simulink model "TBRe_Mod"  (R2017b)
settings: Solver=FixedStepDiscrete  StartTime=0.0  StopTime=inf  FixedStep=0.0001  RelTol=1e-3
PostLoadFcn:
  | model_init();
values from neighbouring files (symbols this model uses):
  SOC_Calc_bPoint = Simulink.Parameter    [ecuparams.m]
  SOC_Calc_Data = Simulink.Parameter    [ecuparams.m]
  Voltage_Act_bPoint = Simulink.Parameter    [ecuparams.m]
  Voltage_Act_Data = Simulink.Parameter    [ecuparams.m]
undefined symbols (not defined in the file or in its folder): _240Nm_Breakpoint, _240Nm_Data, Brake_Active_Threshold, Brk1_OOR_High, Brk1_OOR_Low, Brk2_OOR_High, Brk2_OOR_Low, Motor_To_Road_Speed_Ratio, Throttle_Active_Threshold, Throttle_Torque_Map_
libraries: simulink x26
(part 5 of 8)

== system TBRe_Mod/MainTask/Pre_Processing_Layer/Pedal_Box ==
  note: Non hysteresis brake and throttle bools
  note: Throttle bool and Brake bool are arbitrary values (not rules)
  note: Overall Functionality:
      | - All pedal box sensor values are checked to ensure that they are in the correct voltage range
      | - These sensors are then scaled to be between 0-100 %
      | - APPS Implausibility is performed
      | - Brake pedal implausibility is performed
      | - Thresholds for when brake is considered active, and throttle is considered active are set here (used for RTD and Brake Light activation respectively)
  DAL_Data : Inport
  APPS and BP Plausibility : Subsystem
  APPS_Implausibility_Check : Subsystem
  BPPS_Implausibility_Check : Subsystem
  Brake Bool Hysteresis : Relay  OnSwitchValue=Brake_Active_Threshold  OffSwitchValue=Brake_Active_Threshold/2  OutDataTypeStr=boolean
  Brake Out Of Range Check : Subsystem
  Bus Creator : BusCreator  Inputs=13
  Bus Selector : BusSelector  OutputSignals=DAL_Hardwired.Throttle1_Voltage,DAL_Hardwired.Throttle2_Voltage,DAL_Hardwired.Brake1_Pressure,DAL_Hardwired.Brake2_Pressure
  Memory read : S-Function  Commented=on  FunctionName=NsiMem_Read  Parameters=name_var,type_var,size_var,tunable_var  SFunctionDeploymentMode=off  EnableBusSupport=off  mask(Memory read){name_var=Gearing_Ratio, type_var=Unsigned Byte, size_var=1, tunable_var=on}
      mask prompts: name_var "Variable name :"; type_var "Type :"; size_var "Dim of table :"; tunable_var "Is Tunable By USB?"
      mask help: Reads current value of variable memory declared in the configurator block in calibration page.
      mask init:
      | NsiMem_Read_InitializationFcn();
      settings: OpenFcn=NsiMem_Read_OpenFcn();
      mask Help:
      | eval('block=get_param(gcb, ''RTWdata'');')
      | web([docroot '\toolbox\MUXlink\html\blocks/' block.MUXlink_BlockType '.html'])
      mask TypeOptions name_var: Gearing_Ratio | Wheel_Size | Brake1_High | Brake2_High | Throttle1_High | Throttle2_High | Brake1_Low | Brake2_Low | Throttle1_Low | Throttle2_Low | Max_Torque_Std | Green_TSAL2 | Green_TSAL1 | Max_Torque_Boost | MCU_Ignition | LV_Low_Voltage_Warning | MCUMotor_Temp_Warning | Target_Slip_Ratio | TC_P_Gain | MinTC_Torque | Max_Regen | INV_Torque_limit | INV_Speed_Limit_Fwd | INV_Speed_limit_Rev | INV_DC_Link_Target | INV_DC_Link_Regen_Imax | INV_DC_Link_Discharge_Imax | INV_Regen_Torque_Limit | INV_Id_Debug | INV_Iq_debug | Init_System_Start | Init_System_end | Brake1_Pressure_Scaling | Brake2_Pressure_Scaling | Regen_Coast
      mask Callback name_var: NsiMem_Read_ApplyFcn(1);
      mask TypeOptions type_var: Boolean | Signed Byte | Unsigned Byte | Signed Word | Unsigned Word | Signed Double Word | Unsigned Double Word | Single Float | Double Float
      mask Callback type_var: NsiMem_Read_ApplyFcn(2);
      mask Callback size_var: NsiMem_Read_ApplyFcn(3);
      mask Callback tunable_var: NsiMem_Read_ApplyFcn(4);
      mask Display: image(imread('nsi.bmp'));text(0.5, 0.35, 'Gearing_Ratio', 'horizontalAlignment', 'center', 'verticalAlignment', 'base');plot([0.05 0.05 0.05 0.05 0.05 0.05 0.05 0.05 0.05 0.05]);port_label('output', 1, 'Read');
  Memory read1 : S-Function  Commented=on  FunctionName=NsiMem_Read  Parameters=name_var,type_var,size_var,tunable_var  SFunctionDeploymentMode=off  EnableBusSupport=off  mask(Memory read){name_var=Gearing_Ratio, type_var=Unsigned Byte, size_var=1, tunable_var=on}
      mask prompts: name_var "Variable name :"; type_var "Type :"; size_var "Dim of table :"; tunable_var "Is Tunable By USB?"
      mask help: Reads current value of variable memory declared in the configurator block in calibration page.
      mask init:
      | NsiMem_Read_InitializationFcn();
      settings: OpenFcn=NsiMem_Read_OpenFcn();
      mask Help:
      | eval('block=get_param(gcb, ''RTWdata'');')
      | web([docroot '\toolbox\MUXlink\html\blocks/' block.MUXlink_BlockType '.html'])
      mask TypeOptions name_var: Gearing_Ratio | Wheel_Size | Brake1_High | Brake2_High | Throttle1_High | Throttle2_High | Brake1_Low | Brake2_Low | Throttle1_Low | Throttle2_Low | Max_Torque_Std | Green_TSAL2 | Green_TSAL1 | Max_Torque_Boost | MCU_Ignition | LV_Low_Voltage_Warning | MCUMotor_Temp_Warning | Target_Slip_Ratio | TC_P_Gain | MinTC_Torque | Max_Regen | INV_Torque_limit | INV_Speed_Limit_Fwd | INV_Speed_limit_Rev | INV_DC_Link_Target | INV_DC_Link_Regen_Imax | INV_DC_Link_Discharge_Imax | INV_Regen_Torque_Limit | INV_Id_Debug | INV_Iq_debug | Init_System_Start | Init_System_end | Brake1_Pressure_Scaling | Brake2_Pressure_Scaling | Regen_Coast
      mask Callback name_var: NsiMem_Read_ApplyFcn(1);
      mask TypeOptions type_var: Boolean | Signed Byte | Unsigned Byte | Signed Word | Unsigned Word | Signed Double Word | Unsigned Double Word | Single Float | Double Float
      mask Callback type_var: NsiMem_Read_ApplyFcn(2);
      mask Callback size_var: NsiMem_Read_ApplyFcn(3);
      mask Callback tunable_var: NsiMem_Read_ApplyFcn(4);
      mask Display: image(imread('nsi.bmp'));text(0.5, 0.35, 'Gearing_Ratio', 'horizontalAlignment', 'center', 'verticalAlignment', 'base');plot([0.05 0.05 0.05 0.05 0.05 0.05 0.05 0.05 0.05 0.05]);port_label('output', 1, 'Read');
  Relational Operator : RelationalOperator  Commented=on  OutDataTypeStr=boolean  RndMeth=Simplest
  Relational Operator1 : RelationalOperator  Commented=on  OutDataTypeStr=boolean  RndMeth=Simplest
  Sensor Plausibility : Subsystem
  Throttle Bool Hysteresis : Relay  OnSwitchValue=Throttle_Active_Threshold  OffSwitchValue=Throttle_Active_Threshold/2  OutDataTypeStr=boolean
  Voltage_to_% Conversion : Subsystem
  Pedal_Box_Data : Outport
  wires:
  Bus Creator/1 -> Pedal_Box_Data/1
  DAL_Data/1 -> Brake Out Of Range Check/1(Brake Voltages), Bus Selector/1
  Voltage_to_% Conversion/1(T1%) -> Bus Creator/2, APPS_Implausibility_Check/1(Throttle1_Per)  "Throttle1_Per"
  Voltage_to_% Conversion/2(T2%) -> Bus Creator/3, APPS_Implausibility_Check/2(Throttle2_Per)  "Throttle2_Per"
  Throttle Bool Hysteresis/1 -> Bus Creator/6  "Throttle_Bool"
  Brake Bool Hysteresis/1 -> Bus Creator/8  "Brake_Bool"
  APPS and BP Plausibility/1(Throttle_%) -> Bus Creator/5, Throttle Bool Hysteresis/1  "Throttle_Percentage"
  APPS and BP Plausibility/2(APPS_BP_Implausibility) -> Bus Creator/7  "APPS_BP_Implausibility"
  APPS_Implausibility_Check/1(APPS_Implausibility) -> Bus Creator/4  "APPS_Implausibility"
  APPS_Implausibility_Check/2(Throttle_%) -> APPS and BP Plausibility/1(Throttle_In)
  Sensor Plausibility/1(Pedal_Sensor_Fail) -> Bus Creator/1  "Pedal_Sensor_Fail"
  Bus Selector/1 -> Sensor Plausibility/1(<Throttle1_Voltage>)  "<Throttle1_Voltage>"
  Bus Selector/2 -> Sensor Plausibility/2(<Throttle2_Voltage>)  "<Throttle2_Voltage>"
  Sensor Plausibility/2(TV1_Out) -> Voltage_to_% Conversion/1(Throttle1)
  Sensor Plausibility/3(TV2_Out) -> Voltage_to_% Conversion/2(Throttle2)
  Bus Selector/3 -> Sensor Plausibility/3(<Brake_Voltage>1)  "<Brake1_Pressure>"
  Bus Selector/4 -> Sensor Plausibility/4(<Brake_Voltage>2)  "<Brake2_Pressure>"
  Sensor Plausibility/4(BV1_Out) -> Voltage_to_% Conversion/3(BrakePress1)
  Sensor Plausibility/5(BV1_Out1) -> Voltage_to_% Conversion/4(BrakePress2)
  BPPS_Implausibility_Check/1(Brake_%) -> Brake Bool Hysteresis/1, Bus Creator/9, APPS and BP Plausibility/2(Brake_%)  "Brake_Percentage"
  BPPS_Implausibility_Check/2(BPPS_Implausibility) -> Bus Creator/10  "BPPS_Implausibility"
  Voltage_to_% Conversion/3(BPr%1) -> Bus Creator/11, BPPS_Implausibility_Check/1(Brake1_Per)  "Brake1_Per"
  Voltage_to_% Conversion/4(BPr%2) -> Bus Creator/12, BPPS_Implausibility_Check/2(Brake2_Per)  "Brake2_Per"
  ? -> Relational Operator/1  "Brake_Percentage"
  Memory read1/1 -> Relational Operator/2
  ? -> Relational Operator1/1  "Throttle_Percentage"
  Memory read/1 -> Relational Operator1/2
  Brake Out Of Range Check/1(Brake Out Of Range) -> Bus Creator/13  "Brake_OOR"

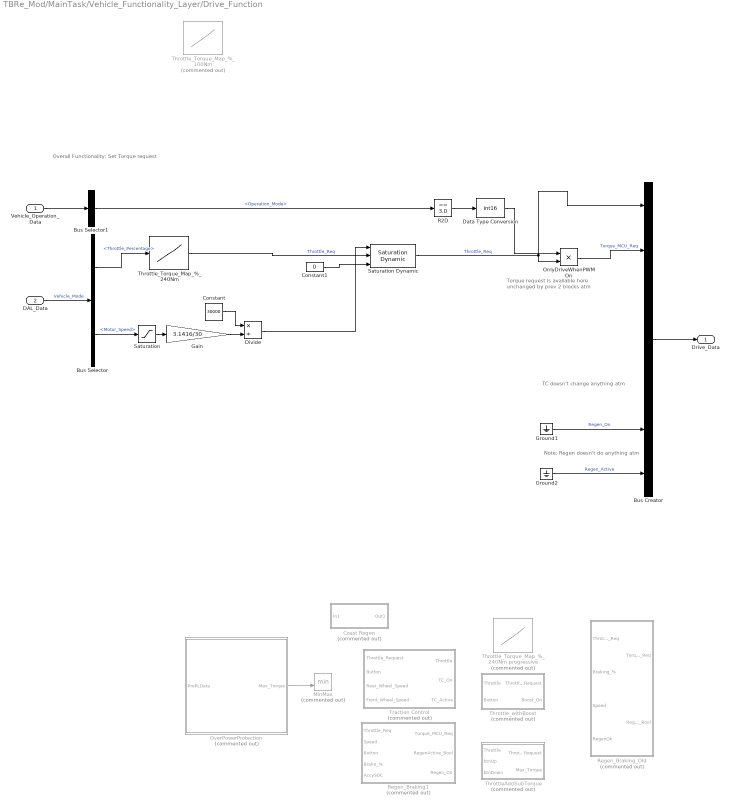
== system TBRe_Mod/MainTask/Vehicle_Functionality_Layer/Drive_Function ==
  note: Torque request is available here
      | unchanged by prev 2 blocks atm
  note: TC doesn't change anything atm
  note: Note: Regen doesn't do anything atm
  note: Overall Functionality:
      | Set Torque request
  Vehicle_Operation_Data : Inport
  DAL_Data : Inport  Port=2
  Bus Creator : BusCreator  Inputs=7
  Bus Selector : BusSelector  OutputSignals=Pedal_Box_Data.Throttle_Percentage,HAL_Data.DAL_CAN.DAL_MCUCAN.Motor_Speed
  Bus Selector1 : BusSelector  OutputSignals=Operation_Mode
  Coast Regen : Subsystem  Commented=on
  Constant : Constant  Value=30000
  Constant1 : Constant  Value=0
  Data Type Conversion : DataTypeConversion  OutDataTypeStr=int16
  Divide : Product  Inputs=*/
  Gain : Gain  Gain=3.1416/30
  Ground1 : Ground
  Ground2 : Ground
  MinMax : MinMax  Commented=on  Inputs=2
  OnlyDriveWhenPWMOn : Product  OutDataTypeStr=int16
  OverPowerProtection : Subsystem  Commented=on
  R2D : simulink/Logic and Bit Operations/Compare To Constant  relop===  const=3.0  OutDataTypeStr=boolean
  Regen_Braking1 : Subsystem  Commented=on
  Regen_Braking_Old : Subsystem  Commented=on
  Saturation : Saturate  UpperLimit=10000  LowerLimit=1
  Saturation Dynamic : simulink/Discontinuities/Saturation Dynamic  OutMin=[]  OutMax=[]  OutDataTypeStr=Inherit: Same as second input  OutDataType=fixdt(1, 16)  OutScaling=2^-10  DoSatur=off
  ThrottleAddSubTorque : Subsystem  Commented=on
  Throttle_Torque_Map_%_100Nm : Lookup_n-D  Commented=on  NumberOfTableDimensions=1  BreakpointsForDimension1=[0,25,100]  Table=[0,10,100]  ExtrapMethod=Clip  UseLastTableValue=on  InternalRulePriority=Speed  OutDataTypeStr=int16  RndMeth=Simplest  InputSameDT=on
  Throttle_Torque_Map_%_240Nm : Lookup_n-D  NumberOfTableDimensions=1  BreakpointsForDimension1=Throttle_Torque_Map_%_240Nm_Breakpoint  Table=Throttle_Torque_Map_%_240Nm_Data  ExtrapMethod=Clip  UseLastTableValue=on  InternalRulePriority=Speed  OutDataTypeStr=int16  RndMeth=Simplest  InputSameDT=on
  Throttle_Torque_Map_%_240Nm progressive : Lookup_n-D  Commented=on  NumberOfTableDimensions=1  BreakpointsForDimension1=[0,10,20,40,60,80,100]  Table=[0,20,30,50,120,200,240]  ExtrapMethod=Clip  UseLastTableValue=on  InternalRulePriority=Speed  OutDataTypeStr=int16  RndMeth=Simplest  InputSameDT=on
  Throttle_withBoost : Subsystem  Commented=on
  Traction Control : Subsystem  Commented=on
  Drive_Data : Outport
  wires:
  Bus Selector1/1 -> R2D/1  "<Operation_Mode>"
  Bus Selector/1 -> Throttle_Torque_Map_%_240Nm/1  "<Throttle_Percentage>"
  R2D/1 -> Data Type Conversion/1
  Vehicle_Operation_Data/1 -> Bus Selector1/1
  DAL_Data/1 -> Bus Selector/1  "Vehicle_Mode"
  OnlyDriveWhenPWMOn/1 -> Bus Creator/2  "Torque_MCU_Req"
  Bus Creator/1 -> Drive_Data/1
  Data Type Conversion/1 -> OnlyDriveWhenPWMOn/1
  Ground1/1 -> Bus Creator/6  "Regen_On"
  OverPowerProtection/1(Max_Torque) -> MinMax/2
  Ground2/1 -> Bus Creator/7  "Regen_Active"
  Saturation Dynamic/1 -> Bus Creator/1, OnlyDriveWhenPWMOn/2  "Throttle_Req"
  Bus Selector/2 -> Saturation/1  "<Motor_Speed>"
  Throttle_Torque_Map_%_240Nm/1 -> Saturation Dynamic/2  "Throttle_Req"
  Gain/1 -> Divide/2
  Constant/1 -> Divide/1
  Divide/1 -> Saturation Dynamic/1
  Constant1/1 -> Saturation Dynamic/3
  Saturation/1 -> Gain/1

== system TBRe_Mod/MainTask/Vehicle_Functionality_Layer/Vehicle_Operation_Mode ==
  note: Checks high contactor has physically closed and request to close is beening sent
  note: System_Error
  note: Overall Functionality:
      | Vehicle state machine for Ready to drive after checking the vehicle is safe,
      | Put vehicel in error state if nessassery
      | Activate TSS
  PrePL_Data : Inport
  Bus Creator : BusCreator  Inputs=6
  Bus Selector1 : BusSelector  OutputSignals=Pedal_Box_Data.Throttle_Bool,Pedal_Box_Data.Brake_Bool,Buttons.btnRTD,HAL_Data.DAL_Hardwired.AIRHigh
  Bus Selector2 : BusSelector  OutputSignals=HAL_Data.DAL_CAN.DAL_SENSORCAN.Shutdown_Error,LV_Battery.LV_Warning,MCU_Temps_Data.MCU_Motor_Temp_Error,Pedal_Box_Data.Brake_OOR,IMD_Data.IMD_Freq
  Bus Selector3 : BusSelector  OutputSignals=HAL_Data.DAL_Hardwired.btnPreCharge_Input,HAL_Data.DAL_Hardwired.AIRLow,HAL_Data.DAL_Hardwired.Latch_Status
  Compare To Constant2 : simulink/Logic and Bit Operations/Compare To Constant  relop=~=  const=0  OutDataTypeStr=boolean
  Logical Operator1 : Logic  AllPortsSameDT=off  OutDataTypeStr=boolean
  Logical Operator2 : Logic  AllPortsSameDT=off  OutDataTypeStr=boolean
  Operaton_Mode : Stateflow chart  TreatAsAtomicUnit=on
  TS Enable : Stateflow chart  TreatAsAtomicUnit=on
  TSS (Precharge Finisher) : Subsystem
  Terminator{1,3..5} (4 alike) : Terminator
  VOM_Data : Outport
  wires:
  Bus Selector1/2 -> Operaton_Mode/2(Brake)  "<Brake_Bool>"
  Logical Operator1/1 -> Bus Creator/3  "ECU_Ok"
  Operaton_Mode/1(Control_Word) -> Bus Creator/1  "Control_Word"
  Operaton_Mode/2(State) -> Compare To Constant2/1, Bus Creator/2  "Operation_Mode"
  Bus Creator/1 -> VOM_Data/1  "Vehicle_Operation_Data"
  Bus Selector1/1 -> Operaton_Mode/1(Throttle)  "<Throttle_Bool>"
  TSS (Precharge Finisher)/1(TS_StartUp) -> Logical Operator2/2, Bus Creator/4  "TSS"
  Bus Selector1/3 -> Operaton_Mode/3(btnRTD)  "<btnRTD>"
  Bus Selector2/3 -> Terminator3/1  "<MCU_Motor_Temp_Error>"
  Bus Selector2/2 -> Terminator5/1  "<LV_Warning>"
  Bus Selector2/1 -> Terminator4/1  "<Shutdown_Error>"
  PrePL_Data/1 -> Bus Selector3/1, TSS (Precharge Finisher)/1(PrePL_Data), Bus Selector2/1, Bus Selector1/1  "Input_Data"
  Bus Selector3/1 -> TS Enable/1(btnPreCharge)  "<btnPreCharge_Input>"
  Bus Selector3/2 -> TS Enable/2(LowAIR_Status)  "<AIRLow>"
  TS Enable/1(TS_Enable) -> Logical Operator1/2, TSS (Precharge Finisher)/2(TS_Enable)
  Compare To Constant2/1 -> Logical Operator1/1
  Bus Selector1/4 -> Logical Operator2/1  "<AIRHigh>"
  TS Enable/2(State) -> Bus Creator/5  "TS_Enable_State"
  Logical Operator2/1 -> Operaton_Mode/5(Discharge_ready)
  Bus Selector3/3 -> TS Enable/4(Latch_Status)  "<Latch_Status>"
  Bus Selector2/4 -> Terminator1/1  "<Brake_OOR>"
  ? -> Bus Creator/6  "Reset_Out"

== system TBRe_Mod/MainTask/Comms_And_Data_Acquisition_Layer/Hardwired_Inputs_2019/AIRs ==
  DigitalInput : S-Function  FunctionName=NsiIo_DigitalInput  Parameters=channel,is_trigger,typeof_trigger,is_wakeup,wakeup_level  SFunctionDeploymentMode=off  EnableBusSupport=off  mask(MUXlink I/O Digital Input){channel=21, is_trigger=off, typeof_trigger=Either, is_wakeup=off, wakeup_level=Low level}
      mask prompts: channel "Channel ?"; is_trigger "Trigger ?"; typeof_trigger "Type of Trigger ?"; is_wakeup "Wake-up ?"; wakeup_level "Wake-up level ?"
      mask help: Read digital input from I/O channel.
      mask init:
      | NsiIo_DigitalInput_InitializationFcn();
      settings: OpenFcn=NsiIo_DigitalInput_OpenFcn();
      mask Help:
      | eval('block=get_param(gcb, ''RTWdata'');')
      | web([docroot '\toolbox\MUXlink\html\blocks/' block.MUXlink_BlockType '.html'])
      mask Callback channel: NsiIo_DigitalInput_ApplyFcn(1);
      mask Callback is_trigger: NsiIo_DigitalInput_ApplyFcn(2);
      mask TypeOptions typeof_trigger: Rising | Falling | Either
      mask Callback typeof_trigger: NsiIo_DigitalInput_ApplyFcn(3);
      mask Callback is_wakeup: NsiIo_DigitalInput_ApplyFcn(4);
      mask TypeOptions wakeup_level: Low level | High level
      mask Callback wakeup_level: NsiIo_DigitalInput_ApplyFcn(5);
      mask Display: image(imread('nsi.bmp'));text(0.5, 0.2, 'DigitalInput_21', 'horizontalAlignment', 'center', 'verticalAlignment', 'base');plot([0.05 0.05 0.05 0.05 0.05 0.05 0.05 0.05 0.05 0.05]);port_label('output', 1, 'Battery : F1');
  DigitalInput5 : S-Function  FunctionName=NsiIo_DigitalInput  Parameters=channel,is_trigger,typeof_trigger,is_wakeup,wakeup_level  SFunctionDeploymentMode=off  EnableBusSupport=off  mask(MUXlink I/O Digital Input){channel=22, is_trigger=off, typeof_trigger=Either, is_wakeup=off, wakeup_level=Low level}
      mask prompts: channel "Channel ?"; is_trigger "Trigger ?"; typeof_trigger "Type of Trigger ?"; is_wakeup "Wake-up ?"; wakeup_level "Wake-up level ?"
      mask help: Read digital input from I/O channel.
      mask init:
      | NsiIo_DigitalInput_InitializationFcn();
      settings: OpenFcn=NsiIo_DigitalInput_OpenFcn();
      mask Help:
      | eval('block=get_param(gcb, ''RTWdata'');')
      | web([docroot '\toolbox\MUXlink\html\blocks/' block.MUXlink_BlockType '.html'])
      mask Callback channel: NsiIo_DigitalInput_ApplyFcn(1);
      mask Callback is_trigger: NsiIo_DigitalInput_ApplyFcn(2);
      mask TypeOptions typeof_trigger: Rising | Falling | Either
      mask Callback typeof_trigger: NsiIo_DigitalInput_ApplyFcn(3);
      mask Callback is_wakeup: NsiIo_DigitalInput_ApplyFcn(4);
      mask TypeOptions wakeup_level: Low level | High level
      mask Callback wakeup_level: NsiIo_DigitalInput_ApplyFcn(5);
      mask Display: image(imread('nsi.bmp'));text(0.5, 0.2, 'DigitalInput_22', 'horizontalAlignment', 'center', 'verticalAlignment', 'base');plot([0.05 0.05 0.05 0.05 0.05 0.05 0.05 0.05 0.05 0.05]);port_label('output', 1, 'Battery : F2');
  UsbTx1 : S-Function  FunctionName=NsiUsb_Tx  Parameters=signame,resolution,offset,unite  SFunctionDeploymentMode=off  EnableBusSupport=off  mask(MUXlink Usb Tx){signame=AIRLow, resolution=1, offset=0, unite=Bool}
      mask prompts: signame "Signal name ?"; resolution "Resolution ?"; offset "Offset ?"; unite "Unit ?"
      mask help: Transmit a frame on the USB Channel.
      mask init:
      | NsiUsb_Tx_InitializationFcn();
      settings: OpenFcn=NsiUsb_Tx_OpenFcn();
      mask Help:
      | eval('block=get_param(gcb, ''RTWdata'');')
      | web([docroot '\toolbox\MUXlink\html\blocks/' block.MUXlink_BlockType '.html'])
      mask Callback signame: NsiUsb_Tx_ApplyFcn(1);
      mask Callback resolution: NsiUsb_Tx_ApplyFcn(2);
      mask Callback offset: NsiUsb_Tx_ApplyFcn(3);
      mask Callback unite: NsiUsb_Tx_ApplyFcn(4);
      mask Display: image(imread('nsi.bmp'));text(0.5, 0.2, 'USB Tx', 'horizontalAlignment', 'center', 'verticalAlignment', 'base');plot([0.05 0.05 0.05 0.05 0.05 0.05 0.05 0.05 0.05 0.05]);port_label('input',1, 'AIRLow');
  UsbTx2 : S-Function  FunctionName=NsiUsb_Tx  Parameters=signame,resolution,offset,unite  SFunctionDeploymentMode=off  EnableBusSupport=off  mask(MUXlink Usb Tx){signame=AIRHigh, resolution=1, offset=0, unite=Bool}
      mask prompts: signame "Signal name ?"; resolution "Resolution ?"; offset "Offset ?"; unite "Unit ?"
      mask help: Transmit a frame on the USB Channel.
      mask init:
      | NsiUsb_Tx_InitializationFcn();
      settings: OpenFcn=NsiUsb_Tx_OpenFcn();
      mask Help:
      | eval('block=get_param(gcb, ''RTWdata'');')
      | web([docroot '\toolbox\MUXlink\html\blocks/' block.MUXlink_BlockType '.html'])
      mask Callback signame: NsiUsb_Tx_ApplyFcn(1);
      mask Callback resolution: NsiUsb_Tx_ApplyFcn(2);
      mask Callback offset: NsiUsb_Tx_ApplyFcn(3);
      mask Callback unite: NsiUsb_Tx_ApplyFcn(4);
      mask Display: image(imread('nsi.bmp'));text(0.5, 0.2, 'USB Tx', 'horizontalAlignment', 'center', 'verticalAlignment', 'base');plot([0.05 0.05 0.05 0.05 0.05 0.05 0.05 0.05 0.05 0.05]);port_label('input',1, 'AIRHigh');
  AIRLow : Outport
  AIRHigh : Outport  Port=2
  wires:
  DigitalInput/1 -> UsbTx1/1, AIRLow/1  "AIRLow"
  DigitalInput5/1 -> UsbTx2/1, AIRHigh/1  "AIRHigh"

== system TBRe_Mod/MainTask/Comms_And_Data_Acquisition_Layer/Hardwired_Inputs_2019/BMS ==
  DigitalInput1 : S-Function  FunctionName=NsiIo_DigitalInput  Parameters=channel,is_trigger,typeof_trigger,is_wakeup,wakeup_level  SFunctionDeploymentMode=off  EnableBusSupport=off  mask(MUXlink I/O Digital Input){channel=16, is_trigger=off, typeof_trigger=Either, is_wakeup=off, wakeup_level=Low level}
      mask prompts: channel "Channel ?"; is_trigger "Trigger ?"; typeof_trigger "Type of Trigger ?"; is_wakeup "Wake-up ?"; wakeup_level "Wake-up level ?"
      mask help: Read digital input from I/O channel.
      mask init:
      | NsiIo_DigitalInput_InitializationFcn();
      settings: OpenFcn=NsiIo_DigitalInput_OpenFcn();
      mask Help:
      | eval('block=get_param(gcb, ''RTWdata'');')
      | web([docroot '\toolbox\MUXlink\html\blocks/' block.MUXlink_BlockType '.html'])
      mask Callback channel: NsiIo_DigitalInput_ApplyFcn(1);
      mask Callback is_trigger: NsiIo_DigitalInput_ApplyFcn(2);
      mask TypeOptions typeof_trigger: Rising | Falling | Either
      mask Callback typeof_trigger: NsiIo_DigitalInput_ApplyFcn(3);
      mask Callback is_wakeup: NsiIo_DigitalInput_ApplyFcn(4);
      mask TypeOptions wakeup_level: Low level | High level
      mask Callback wakeup_level: NsiIo_DigitalInput_ApplyFcn(5);
      mask Display: image(imread('nsi.bmp'));text(0.5, 0.2, 'DigitalInput_16', 'horizontalAlignment', 'center', 'verticalAlignment', 'base');plot([0.05 0.05 0.05 0.05 0.05 0.05 0.05 0.05 0.05 0.05]);port_label('output', 1, 'Battery : H2');
  DigitalInput2 : S-Function  FunctionName=NsiIo_DigitalInput  Parameters=channel,is_trigger,typeof_trigger,is_wakeup,wakeup_level  SFunctionDeploymentMode=off  EnableBusSupport=off  mask(MUXlink I/O Digital Input){channel=17, is_trigger=off, typeof_trigger=Either, is_wakeup=off, wakeup_level=Low level}
      mask prompts: channel "Channel ?"; is_trigger "Trigger ?"; typeof_trigger "Type of Trigger ?"; is_wakeup "Wake-up ?"; wakeup_level "Wake-up level ?"
      mask help: Read digital input from I/O channel.
      mask init:
      | NsiIo_DigitalInput_InitializationFcn();
      settings: OpenFcn=NsiIo_DigitalInput_OpenFcn();
      mask Help:
      | eval('block=get_param(gcb, ''RTWdata'');')
      | web([docroot '\toolbox\MUXlink\html\blocks/' block.MUXlink_BlockType '.html'])
      mask Callback channel: NsiIo_DigitalInput_ApplyFcn(1);
      mask Callback is_trigger: NsiIo_DigitalInput_ApplyFcn(2);
      mask TypeOptions typeof_trigger: Rising | Falling | Either
      mask Callback typeof_trigger: NsiIo_DigitalInput_ApplyFcn(3);
      mask Callback is_wakeup: NsiIo_DigitalInput_ApplyFcn(4);
      mask TypeOptions wakeup_level: Low level | High level
      mask Callback wakeup_level: NsiIo_DigitalInput_ApplyFcn(5);
      mask Display: image(imread('nsi.bmp'));text(0.5, 0.2, 'DigitalInput_17', 'horizontalAlignment', 'center', 'verticalAlignment', 'base');plot([0.05 0.05 0.05 0.05 0.05 0.05 0.05 0.05 0.05 0.05]);port_label('output', 1, 'Battery : H3');
  DigitalInput6 : S-Function  FunctionName=NsiIo_DigitalInput  Parameters=channel,is_trigger,typeof_trigger,is_wakeup,wakeup_level  SFunctionDeploymentMode=off  EnableBusSupport=off  mask(MUXlink I/O Digital Input){channel=18, is_trigger=off, typeof_trigger=Either, is_wakeup=off, wakeup_level=Low level}
      mask prompts: channel "Channel ?"; is_trigger "Trigger ?"; typeof_trigger "Type of Trigger ?"; is_wakeup "Wake-up ?"; wakeup_level "Wake-up level ?"
      mask help: Read digital input from I/O channel.
      mask init:
      | NsiIo_DigitalInput_InitializationFcn();
      settings: OpenFcn=NsiIo_DigitalInput_OpenFcn();
      mask Help:
      | eval('block=get_param(gcb, ''RTWdata'');')
      | web([docroot '\toolbox\MUXlink\html\blocks/' block.MUXlink_BlockType '.html'])
      mask Callback channel: NsiIo_DigitalInput_ApplyFcn(1);
      mask Callback is_trigger: NsiIo_DigitalInput_ApplyFcn(2);
      mask TypeOptions typeof_trigger: Rising | Falling | Either
      mask Callback typeof_trigger: NsiIo_DigitalInput_ApplyFcn(3);
      mask Callback is_wakeup: NsiIo_DigitalInput_ApplyFcn(4);
      mask TypeOptions wakeup_level: Low level | High level
      mask Callback wakeup_level: NsiIo_DigitalInput_ApplyFcn(5);
      mask Display: image(imread('nsi.bmp'));text(0.5, 0.2, 'DigitalInput_18', 'horizontalAlignment', 'center', 'verticalAlignment', 'base');plot([0.05 0.05 0.05 0.05 0.05 0.05 0.05 0.05 0.05 0.05]);port_label('output', 1, 'Battery : H4');
  BMS_Multi1 : Outport
  BMS_Multi2 : Outport  Port=2
  BMS_ChargeEnable : Outport  Port=3
  wires:
  DigitalInput6/1 -> BMS_Multi1/1  "BMS_Multi1"
  DigitalInput2/1 -> BMS_ChargeEnable/1  "BMS_ChargeEnable"
  DigitalInput1/1 -> BMS_Multi2/1  "BMS_Multi2"

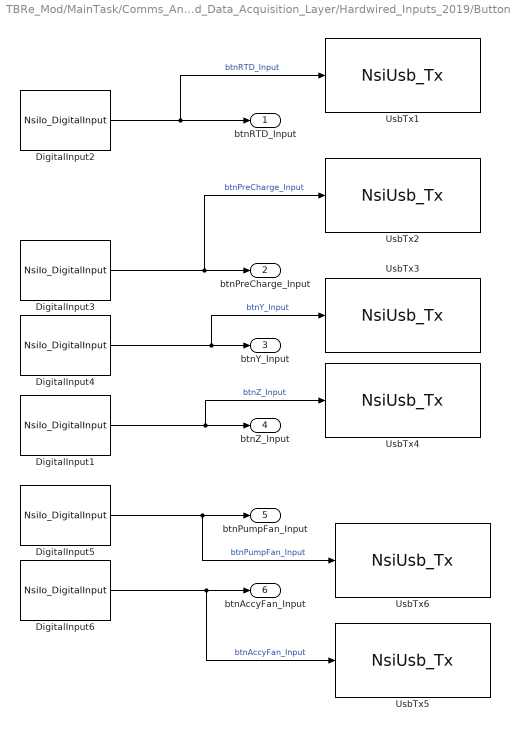
== system TBRe_Mod/MainTask/Comms_And_Data_Acquisition_Layer/Hardwired_Inputs_2019/Buttons ==
  DigitalInput1 : S-Function  FunctionName=NsiIo_DigitalInput  Parameters=channel,is_trigger,typeof_trigger,is_wakeup,wakeup_level  SFunctionDeploymentMode=off  EnableBusSupport=off  mask(MUXlink I/O Digital Input){channel=14, is_trigger=off, typeof_trigger=Either, is_wakeup=off, wakeup_level=Low level}
      mask prompts: channel "Channel ?"; is_trigger "Trigger ?"; typeof_trigger "Type of Trigger ?"; is_wakeup "Wake-up ?"; wakeup_level "Wake-up level ?"
      mask help: Read digital input from I/O channel.
      mask init:
      | NsiIo_DigitalInput_InitializationFcn();
      settings: OpenFcn=NsiIo_DigitalInput_OpenFcn();
      mask Help:
      | eval('block=get_param(gcb, ''RTWdata'');')
      | web([docroot '\toolbox\MUXlink\html\blocks/' block.MUXlink_BlockType '.html'])
      mask Callback channel: NsiIo_DigitalInput_ApplyFcn(1);
      mask Callback is_trigger: NsiIo_DigitalInput_ApplyFcn(2);
      mask TypeOptions typeof_trigger: Rising | Falling | Either
      mask Callback typeof_trigger: NsiIo_DigitalInput_ApplyFcn(3);
      mask Callback is_wakeup: NsiIo_DigitalInput_ApplyFcn(4);
      mask TypeOptions wakeup_level: Low level | High level
      mask Callback wakeup_level: NsiIo_DigitalInput_ApplyFcn(5);
      mask Display: image(imread('nsi.bmp'));text(0.5, 0.2, 'DigitalInput_14', 'horizontalAlignment', 'center', 'verticalAlignment', 'base');plot([0.05 0.05 0.05 0.05 0.05 0.05 0.05 0.05 0.05 0.05]);port_label('output', 1, 'Battery : G4');
  DigitalInput2 : S-Function  FunctionName=NsiIo_DigitalInput  Parameters=channel,is_trigger,typeof_trigger,is_wakeup,wakeup_level  SFunctionDeploymentMode=off  EnableBusSupport=off  mask(MUXlink I/O Digital Input){channel=11, is_trigger=off, typeof_trigger=Either, is_wakeup=off, wakeup_level=Low level}
      mask prompts: channel "Channel ?"; is_trigger "Trigger ?"; typeof_trigger "Type of Trigger ?"; is_wakeup "Wake-up ?"; wakeup_level "Wake-up level ?"
      mask help: Read digital input from I/O channel.
      mask init:
      | NsiIo_DigitalInput_InitializationFcn();
      settings: OpenFcn=NsiIo_DigitalInput_OpenFcn();
      mask Help:
      | eval('block=get_param(gcb, ''RTWdata'');')
      | web([docroot '\toolbox\MUXlink\html\blocks/' block.MUXlink_BlockType '.html'])
      mask Callback channel: NsiIo_DigitalInput_ApplyFcn(1);
      mask Callback is_trigger: NsiIo_DigitalInput_ApplyFcn(2);
      mask TypeOptions typeof_trigger: Rising | Falling | Either
      mask Callback typeof_trigger: NsiIo_DigitalInput_ApplyFcn(3);
      mask Callback is_wakeup: NsiIo_DigitalInput_ApplyFcn(4);
      mask TypeOptions wakeup_level: Low level | High level
      mask Callback wakeup_level: NsiIo_DigitalInput_ApplyFcn(5);
      mask Display: image(imread('nsi.bmp'));text(0.5, 0.2, 'DigitalInput_11', 'horizontalAlignment', 'center', 'verticalAlignment', 'base');plot([0.05 0.05 0.05 0.05 0.05 0.05 0.05 0.05 0.05 0.05]);port_label('output', 1, 'Battery : G1');
  DigitalInput3 : S-Function  FunctionName=NsiIo_DigitalInput  Parameters=channel,is_trigger,typeof_trigger,is_wakeup,wakeup_level  SFunctionDeploymentMode=off  EnableBusSupport=off  mask(MUXlink I/O Digital Input){channel=12, is_trigger=off, typeof_trigger=Either, is_wakeup=off, wakeup_level=Low level}
      mask prompts: channel "Channel ?"; is_trigger "Trigger ?"; typeof_trigger "Type of Trigger ?"; is_wakeup "Wake-up ?"; wakeup_level "Wake-up level ?"
      mask help: Read digital input from I/O channel.
      mask init:
      | NsiIo_DigitalInput_InitializationFcn();
      settings: OpenFcn=NsiIo_DigitalInput_OpenFcn();
      mask Help:
      | eval('block=get_param(gcb, ''RTWdata'');')
      | web([docroot '\toolbox\MUXlink\html\blocks/' block.MUXlink_BlockType '.html'])
      mask Callback channel: NsiIo_DigitalInput_ApplyFcn(1);
      mask Callback is_trigger: NsiIo_DigitalInput_ApplyFcn(2);
      mask TypeOptions typeof_trigger: Rising | Falling | Either
      mask Callback typeof_trigger: NsiIo_DigitalInput_ApplyFcn(3);
      mask Callback is_wakeup: NsiIo_DigitalInput_ApplyFcn(4);
      mask TypeOptions wakeup_level: Low level | High level
      mask Callback wakeup_level: NsiIo_DigitalInput_ApplyFcn(5);
      mask Display: image(imread('nsi.bmp'));text(0.5, 0.2, 'DigitalInput_12', 'horizontalAlignment', 'center', 'verticalAlignment', 'base');plot([0.05 0.05 0.05 0.05 0.05 0.05 0.05 0.05 0.05 0.05]);port_label('output', 1, 'Battery : G2');
  DigitalInput4 : S-Function  FunctionName=NsiIo_DigitalInput  Parameters=channel,is_trigger,typeof_trigger,is_wakeup,wakeup_level  SFunctionDeploymentMode=off  EnableBusSupport=off  mask(MUXlink I/O Digital Input){channel=13, is_trigger=off, typeof_trigger=Either, is_wakeup=off, wakeup_level=Low level}
      mask prompts: channel "Channel ?"; is_trigger "Trigger ?"; typeof_trigger "Type of Trigger ?"; is_wakeup "Wake-up ?"; wakeup_level "Wake-up level ?"
      mask help: Read digital input from I/O channel.
      mask init:
      | NsiIo_DigitalInput_InitializationFcn();
      settings: OpenFcn=NsiIo_DigitalInput_OpenFcn();
      mask Help:
      | eval('block=get_param(gcb, ''RTWdata'');')
      | web([docroot '\toolbox\MUXlink\html\blocks/' block.MUXlink_BlockType '.html'])
      mask Callback channel: NsiIo_DigitalInput_ApplyFcn(1);
      mask Callback is_trigger: NsiIo_DigitalInput_ApplyFcn(2);
      mask TypeOptions typeof_trigger: Rising | Falling | Either
      mask Callback typeof_trigger: NsiIo_DigitalInput_ApplyFcn(3);
      mask Callback is_wakeup: NsiIo_DigitalInput_ApplyFcn(4);
      mask TypeOptions wakeup_level: Low level | High level
      mask Callback wakeup_level: NsiIo_DigitalInput_ApplyFcn(5);
      mask Display: image(imread('nsi.bmp'));text(0.5, 0.2, 'DigitalInput_13', 'horizontalAlignment', 'center', 'verticalAlignment', 'base');plot([0.05 0.05 0.05 0.05 0.05 0.05 0.05 0.05 0.05 0.05]);port_label('output', 1, 'Battery : G3');
  DigitalInput5 : S-Function  FunctionName=NsiIo_DigitalInput  Parameters=channel,is_trigger,typeof_trigger,is_wakeup,wakeup_level  SFunctionDeploymentMode=off  EnableBusSupport=off  mask(MUXlink I/O Digital Input){channel=9, is_trigger=off, typeof_trigger=Either, is_wakeup=off, wakeup_level=Low level}
      mask prompts: channel "Channel ?"; is_trigger "Trigger ?"; typeof_trigger "Type of Trigger ?"; is_wakeup "Wake-up ?"; wakeup_level "Wake-up level ?"
      mask help: Read digital input from I/O channel.
      mask init:
      | NsiIo_DigitalInput_InitializationFcn();
      settings: OpenFcn=NsiIo_DigitalInput_OpenFcn();
      mask Help:
      | eval('block=get_param(gcb, ''RTWdata'');')
      | web([docroot '\toolbox\MUXlink\html\blocks/' block.MUXlink_BlockType '.html'])
      mask Callback channel: NsiIo_DigitalInput_ApplyFcn(1);
      mask Callback is_trigger: NsiIo_DigitalInput_ApplyFcn(2);
      mask TypeOptions typeof_trigger: Rising | Falling | Either
      mask Callback typeof_trigger: NsiIo_DigitalInput_ApplyFcn(3);
      mask Callback is_wakeup: NsiIo_DigitalInput_ApplyFcn(4);
      mask TypeOptions wakeup_level: Low level | High level
      mask Callback wakeup_level: NsiIo_DigitalInput_ApplyFcn(5);
      mask Display: image(imread('nsi.bmp'));text(0.5, 0.2, 'DigitalInput_9', 'horizontalAlignment', 'center', 'verticalAlignment', 'base');plot([0.05 0.05 0.05 0.05 0.05 0.05 0.05 0.05 0.05 0.05]);port_label('output', 1, 'Ground : C1');
  DigitalInput6 : S-Function  FunctionName=NsiIo_DigitalInput  Parameters=channel,is_trigger,typeof_trigger,is_wakeup,wakeup_level  SFunctionDeploymentMode=off  EnableBusSupport=off  mask(MUXlink I/O Digital Input){channel=10, is_trigger=off, typeof_trigger=Either, is_wakeup=off, wakeup_level=Low level}
      mask prompts: channel "Channel ?"; is_trigger "Trigger ?"; typeof_trigger "Type of Trigger ?"; is_wakeup "Wake-up ?"; wakeup_level "Wake-up level ?"
      mask help: Read digital input from I/O channel.
      mask init:
      | NsiIo_DigitalInput_InitializationFcn();
      settings: OpenFcn=NsiIo_DigitalInput_OpenFcn();
      mask Help:
      | eval('block=get_param(gcb, ''RTWdata'');')
      | web([docroot '\toolbox\MUXlink\html\blocks/' block.MUXlink_BlockType '.html'])
      mask Callback channel: NsiIo_DigitalInput_ApplyFcn(1);
      mask Callback is_trigger: NsiIo_DigitalInput_ApplyFcn(2);
      mask TypeOptions typeof_trigger: Rising | Falling | Either
      mask Callback typeof_trigger: NsiIo_DigitalInput_ApplyFcn(3);
      mask Callback is_wakeup: NsiIo_DigitalInput_ApplyFcn(4);
      mask TypeOptions wakeup_level: Low level | High level
      mask Callback wakeup_level: NsiIo_DigitalInput_ApplyFcn(5);
      mask Display: image(imread('nsi.bmp'));text(0.5, 0.2, 'DigitalInput_10', 'horizontalAlignment', 'center', 'verticalAlignment', 'base');plot([0.05 0.05 0.05 0.05 0.05 0.05 0.05 0.05 0.05 0.05]);port_label('output', 1, 'Ground : C2');
  UsbTx1 : S-Function  FunctionName=NsiUsb_Tx  Parameters=signame,resolution,offset,unite  SFunctionDeploymentMode=off  EnableBusSupport=off  mask(MUXlink Usb Tx){signame=rtd, resolution=1, offset=0, unite=km/h}
      mask prompts: signame "Signal name ?"; resolution "Resolution ?"; offset "Offset ?"; unite "Unit ?"
      mask help: Transmit a frame on the USB Channel.
      mask init:
      | NsiUsb_Tx_InitializationFcn();
      settings: OpenFcn=NsiUsb_Tx_OpenFcn();
      mask Help:
      | eval('block=get_param(gcb, ''RTWdata'');')
      | web([docroot '\toolbox\MUXlink\html\blocks/' block.MUXlink_BlockType '.html'])
      mask Callback signame: NsiUsb_Tx_ApplyFcn(1);
      mask Callback resolution: NsiUsb_Tx_ApplyFcn(2);
      mask Callback offset: NsiUsb_Tx_ApplyFcn(3);
      mask Callback unite: NsiUsb_Tx_ApplyFcn(4);
      mask Display: image(imread('nsi.bmp'));text(0.5, 0.2, 'USB Tx', 'horizontalAlignment', 'center', 'verticalAlignment', 'base');plot([0.05 0.05 0.05 0.05 0.05 0.05 0.05 0.05 0.05 0.05]);port_label('input',1, 'rtd');
  UsbTx2 : S-Function  FunctionName=NsiUsb_Tx  Parameters=signame,resolution,offset,unite  SFunctionDeploymentMode=off  EnableBusSupport=off  mask(MUXlink Usb Tx){signame=x, resolution=1, offset=0, unite=km/h}
      mask prompts: signame "Signal name ?"; resolution "Resolution ?"; offset "Offset ?"; unite "Unit ?"
      mask help: Transmit a frame on the USB Channel.
      mask init:
      | NsiUsb_Tx_InitializationFcn();
      settings: OpenFcn=NsiUsb_Tx_OpenFcn();
      mask Help:
      | eval('block=get_param(gcb, ''RTWdata'');')
      | web([docroot '\toolbox\MUXlink\html\blocks/' block.MUXlink_BlockType '.html'])
      mask Callback signame: NsiUsb_Tx_ApplyFcn(1);
      mask Callback resolution: NsiUsb_Tx_ApplyFcn(2);
      mask Callback offset: NsiUsb_Tx_ApplyFcn(3);
      mask Callback unite: NsiUsb_Tx_ApplyFcn(4);
      mask Display: image(imread('nsi.bmp'));text(0.5, 0.2, 'USB Tx', 'horizontalAlignment', 'center', 'verticalAlignment', 'base');plot([0.05 0.05 0.05 0.05 0.05 0.05 0.05 0.05 0.05 0.05]);port_label('input',1, 'x');
  UsbTx3 : S-Function  FunctionName=NsiUsb_Tx  Parameters=signame,resolution,offset,unite  SFunctionDeploymentMode=off  EnableBusSupport=off  mask(MUXlink Usb Tx){signame=y, resolution=1, offset=0, unite=km/h}
      mask prompts: signame "Signal name ?"; resolution "Resolution ?"; offset "Offset ?"; unite "Unit ?"
      mask help: Transmit a frame on the USB Channel.
      mask init:
      | NsiUsb_Tx_InitializationFcn();
      settings: OpenFcn=NsiUsb_Tx_OpenFcn();
      mask Help:
      | eval('block=get_param(gcb, ''RTWdata'');')
      | web([docroot '\toolbox\MUXlink\html\blocks/' block.MUXlink_BlockType '.html'])
      mask Callback signame: NsiUsb_Tx_ApplyFcn(1);
      mask Callback resolution: NsiUsb_Tx_ApplyFcn(2);
      mask Callback offset: NsiUsb_Tx_ApplyFcn(3);
      mask Callback unite: NsiUsb_Tx_ApplyFcn(4);
      mask Display: image(imread('nsi.bmp'));text(0.5, 0.2, 'USB Tx', 'horizontalAlignment', 'center', 'verticalAlignment', 'base');plot([0.05 0.05 0.05 0.05 0.05 0.05 0.05 0.05 0.05 0.05]);port_label('input',1, 'y');
  UsbTx4 : S-Function  FunctionName=NsiUsb_Tx  Parameters=signame,resolution,offset,unite  SFunctionDeploymentMode=off  EnableBusSupport=off  mask(MUXlink Usb Tx){signame=z, resolution=1, offset=0, unite=km/h}
      mask prompts: signame "Signal name ?"; resolution "Resolution ?"; offset "Offset ?"; unite "Unit ?"
      mask help: Transmit a frame on the USB Channel.
      mask init:
      | NsiUsb_Tx_InitializationFcn();
      settings: OpenFcn=NsiUsb_Tx_OpenFcn();
      mask Help:
      | eval('block=get_param(gcb, ''RTWdata'');')
      | web([docroot '\toolbox\MUXlink\html\blocks/' block.MUXlink_BlockType '.html'])
      mask Callback signame: NsiUsb_Tx_ApplyFcn(1);
      mask Callback resolution: NsiUsb_Tx_ApplyFcn(2);
      mask Callback offset: NsiUsb_Tx_ApplyFcn(3);
      mask Callback unite: NsiUsb_Tx_ApplyFcn(4);
      mask Display: image(imread('nsi.bmp'));text(0.5, 0.2, 'USB Tx', 'horizontalAlignment', 'center', 'verticalAlignment', 'base');plot([0.05 0.05 0.05 0.05 0.05 0.05 0.05 0.05 0.05 0.05]);port_label('input',1, 'z');
  UsbTx5 : S-Function  FunctionName=NsiUsb_Tx  Parameters=signame,resolution,offset,unite  SFunctionDeploymentMode=off  EnableBusSupport=off  mask(MUXlink Usb Tx){signame=Accy_Fan_swtich, resolution=1, offset=0, unite=bool}
      mask prompts: signame "Signal name ?"; resolution "Resolution ?"; offset "Offset ?"; unite "Unit ?"
      mask help: Transmit a frame on the USB Channel.
      mask init:
      | NsiUsb_Tx_InitializationFcn();
      settings: OpenFcn=NsiUsb_Tx_OpenFcn();
      mask Help:
      | eval('block=get_param(gcb, ''RTWdata'');')
      | web([docroot '\toolbox\MUXlink\html\blocks/' block.MUXlink_BlockType '.html'])
      mask Callback signame: NsiUsb_Tx_ApplyFcn(1);
      mask Callback resolution: NsiUsb_Tx_ApplyFcn(2);
      mask Callback offset: NsiUsb_Tx_ApplyFcn(3);
      mask Callback unite: NsiUsb_Tx_ApplyFcn(4);
      mask Display: image(imread('nsi.bmp'));text(0.5, 0.2, 'USB Tx', 'horizontalAlignment', 'center', 'verticalAlignment', 'base');plot([0.05 0.05 0.05 0.05 0.05 0.05 0.05 0.05 0.05 0.05]);port_label('input',1, 'Accy_Fan_swtich');
  UsbTx6 : S-Function  FunctionName=NsiUsb_Tx  Parameters=signame,resolution,offset,unite  SFunctionDeploymentMode=off  EnableBusSupport=off  mask(MUXlink Usb Tx){signame=PumpAndFan_swtich, resolution=1, offset=0, unite=bool}
      mask prompts: signame "Signal name ?"; resolution "Resolution ?"; offset "Offset ?"; unite "Unit ?"
      mask help: Transmit a frame on the USB Channel.
      mask init:
      | NsiUsb_Tx_InitializationFcn();
      settings: OpenFcn=NsiUsb_Tx_OpenFcn();
      mask Help:
      | eval('block=get_param(gcb, ''RTWdata'');')
      | web([docroot '\toolbox\MUXlink\html\blocks/' block.MUXlink_BlockType '.html'])
      mask Callback signame: NsiUsb_Tx_ApplyFcn(1);
      mask Callback resolution: NsiUsb_Tx_ApplyFcn(2);
      mask Callback offset: NsiUsb_Tx_ApplyFcn(3);
      mask Callback unite: NsiUsb_Tx_ApplyFcn(4);
      mask Display: image(imread('nsi.bmp'));text(0.5, 0.2, 'USB Tx', 'horizontalAlignment', 'center', 'verticalAlignment', 'base');plot([0.05 0.05 0.05 0.05 0.05 0.05 0.05 0.05 0.05 0.05]);port_label('input',1, 'PumpAndFan_swtich');
  btnRTD_Input : Outport
  btnPreCharge_Input : Outport  Port=2
  btnY_Input : Outport  Port=3
  btnZ_Input : Outport  Port=4
  btnPumpFan_Input : Outport  Port=5
  btnAccyFan_Input : Outport  Port=6
  wires:
  DigitalInput2/1 -> UsbTx1/1, btnRTD_Input/1  "btnRTD_Input"
  DigitalInput4/1 -> UsbTx3/1, btnY_Input/1  "btnY_Input"
  DigitalInput3/1 -> UsbTx2/1, btnPreCharge_Input/1  "btnPreCharge_Input"
  DigitalInput1/1 -> UsbTx4/1, btnZ_Input/1  "btnZ_Input"
  DigitalInput5/1 -> UsbTx6/1, btnPumpFan_Input/1  "btnPumpFan_Input"
  DigitalInput6/1 -> UsbTx5/1, btnAccyFan_Input/1  "btnAccyFan_Input"

== system TBRe_Mod/MainTask/Comms_And_Data_Acquisition_Layer/Hardwired_Inputs_2019/IMD ==
  Add : Sum  Inputs=-+
  Constant : Constant  Value=1000
  Constant1 : Constant  Value=100
  Divide : Product  Inputs=*/
  FrequentialInput2 : S-Function  FunctionName=NsiIo_FrequencyInput  Parameters=channel,max_freq,is_digital_input,DutyCycle,MUXlabType  SFunctionDeploymentMode=off  EnableBusSupport=off  mask(MUXlink I/O Frequential Input){channel=1, max_freq=10KHZ, is_digital_input=off, DutyCycle=off, MUXlabType=0}
      mask prompts: max_freq "Max Frequency"; is_digital_input "Used as Digital Input"; DutyCycle "Duty Cycle"; MUXlabType "MUXlab Type"
      mask help: Read Frequency from I/O Frequential Input.
      mask init:
      | NsiIo_FrequencyInput_InitializationFcn();
      settings: OpenFcn=NsiIo_FrequencyInput_OpenFcn();
      mask Help:
      | eval('block=get_param(gcb, ''RTWdata'');')
      | web([docroot '\toolbox\MUXlink\html\blocks/' block.MUXlink_BlockType '.html'])
      mask Callback channel: NsiIo_FrequencyInput_ApplyFcn(1);
      mask TypeOptions max_freq: 10KHZ | 100KHZ
      mask Callback max_freq: NsiIo_FrequencyInput_ApplyFcn(2);
      mask Callback is_digital_input: NsiIo_FrequencyInput_ApplyFcn(3);
      mask Callback DutyCycle: NsiIo_FrequencyInput_ApplyFcn(4);
      mask Display: image(imread('nsi.bmp'));text(0.5, 0.2, 'FrequencyInput_1  10KHZ', 'horizontalAlignment', 'center', 'verticalAlignment', 'base');plot([0.05 0.05 0.05 0.05 0.05 0.05 0.05 0.05 0.05 0.05]);port_label('output', 1, 'Freq C1');
  FrequentialInput3 : S-Function  FunctionName=NsiIo_FrequencyInput  Parameters=channel,max_freq,is_digital_input,DutyCycle,MUXlabType  SFunctionDeploymentMode=off  EnableBusSupport=off  mask(MUXlink I/O Frequential Input){channel=2, max_freq=10KHZ, is_digital_input=off, DutyCycle=on, MUXlabType=0}
      mask prompts: max_freq "Max Frequency"; is_digital_input "Used as Digital Input"; DutyCycle "Duty Cycle"; MUXlabType "MUXlab Type"
      mask help: Read Frequency from I/O Frequential Input.
      mask init:
      | NsiIo_FrequencyInput_InitializationFcn();
      settings: OpenFcn=NsiIo_FrequencyInput_OpenFcn();
      mask Help:
      | eval('block=get_param(gcb, ''RTWdata'');')
      | web([docroot '\toolbox\MUXlink\html\blocks/' block.MUXlink_BlockType '.html'])
      mask Callback channel: NsiIo_FrequencyInput_ApplyFcn(1);
      mask TypeOptions max_freq: 10KHZ | 100KHZ
      mask Callback max_freq: NsiIo_FrequencyInput_ApplyFcn(2);
      mask Callback is_digital_input: NsiIo_FrequencyInput_ApplyFcn(3);
      mask Callback DutyCycle: NsiIo_FrequencyInput_ApplyFcn(4);
      mask Display: image(imread('nsi.bmp'));text(0.5, 0.2, 'FrequencyInput_2  10KHZ', 'horizontalAlignment', 'center', 'verticalAlignment', 'base');plot([0.05 0.05 0.05 0.05 0.05 0.05 0.05 0.05 0.05 0.05]);port_label('output', 1, 'Duty_Cycle C2');
  IMD Freq : Outport
  IMD Duty : Outport  Port=2
  wires:
  FrequentialInput2/1 -> IMD Freq/1  "IMD_Freq"
  FrequentialInput3/1 -> Divide/1  "IMD_Duty"
  Constant/1 -> Divide/2
  Divide/1 -> Add/1
  Constant1/1 -> Add/2
  Add/1 -> IMD Duty/1  "IMD_Duty"
